simulink model "PE"  (R2024a)
settings: Solver=VariableStepAuto  StartTime=0.0  StopTime=1  RelTol=1e-3
InitFcn:
  | Pe=1/25000
  | w=32.2
  | V=8
  | L=150e-6
  | C=220e-6
  | R=3.2
libraries: spsSeriesRLCBranchLib x5, spsDiodeLib x5, spsMeanLib x2, spsVoltageMeasurementLib x2, spsCurrentMeasurementLib x2, spsIGBTDiodeLib x1, spsACVoltageSourceLib x1, spsDCVoltageSourceLib x1, sps_lib x1
settings Model: Creator=mxf1547  LastModifiedBy=mxf1547

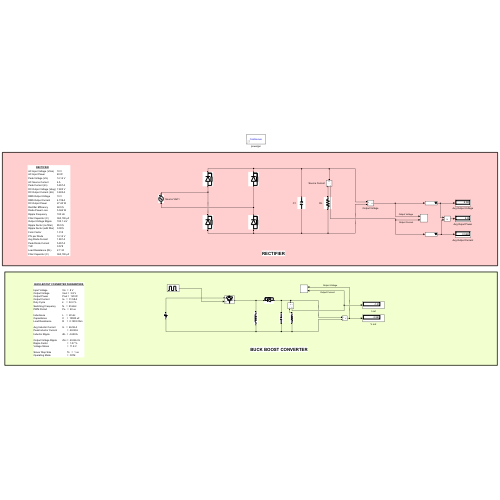
[thumbnail: Simulink's stored preview of the top-level diagram]
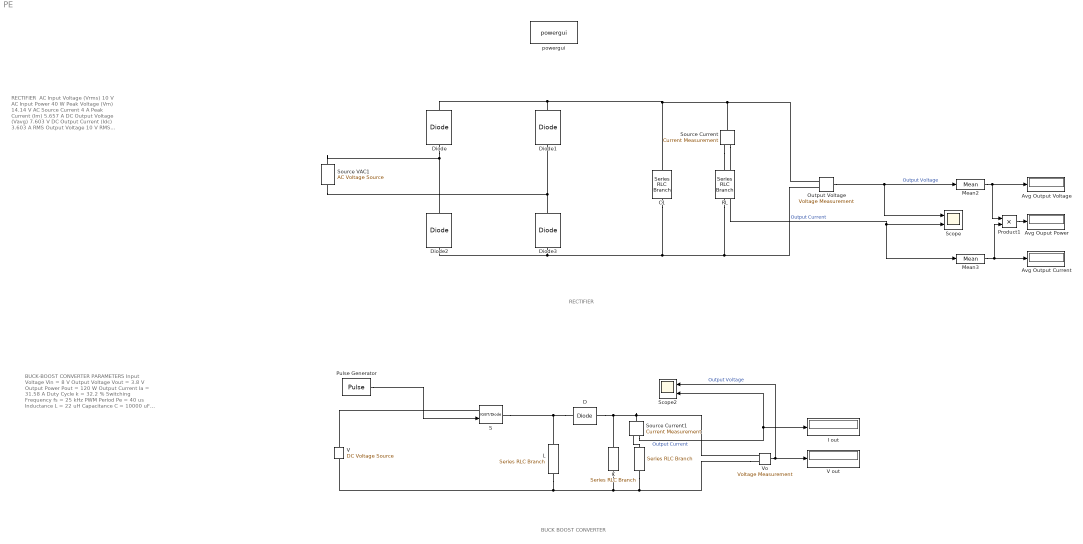
== system PE ==
  note: BUCK-BOOST CONVERTER PARAMETERS
      |
      | Input Voltage Vin = 8 V
      | Output Voltage Vout = 3.8 V
      | Output Power Pout = 120 W
      | Output Current Ia = 31.58 A
      | Duty Cycle k = 32.2 %
      | Switching Frequency fs = 25 kHz
      | PWM Period Pe = 40 us
      |
      | Inductance L = 22 uH
      | Capacitance C = 10000 uF
      | Load Resistance R = 0.1203 Ohm
      |
      | Avg Inductor Current IL = 46.58 A
      | Peak Inductor Current = 48.92 A
      | Inductor Ripple dIL = 4.683 A
      |
      | Output Voltage Ripple dVc = 40.68 mV
      | Ripple Factor = 1.07 %
      | Voltage Stress = 11.8 V
      |
      | Solver Step Size Ts = 1 us
      | Operating Mode = CCM
  note: RECTIFIER
  note: BUCK BOOST CONVERTER
  note: RECTIFIER
      | ​
      |
      | AC Input Voltage (Vrms​)
      | 10 V
      |
      | AC Input Power
      | 40 W
      |
      | Peak Voltage (Vm​)
      | 14.14 V
      |
      | AC Source Current
      | 4 A
      |
      | Peak Current (Im​)
      | 5.657 A
      |
      | DC Output Voltage (Vavg​)
      | 7.603 V
      |
      | DC Output Current (Idc​)
      | 3.603 A
      |
      | RMS Output Voltage
      | 10 V
      |
      | RMS Output Current
      | 4.739 A
      |
      | DC Output Power
      | 27.40 W
      |
      | Rectifier Efficiency
      | 68.5%
      |
      | Diode Power Loss
      | 5.044 W
      |
      | Ripple Frequency
      | 100 Hz
      |
      | Filter Capacitor (C)
      | 360,100 μF
      |
      | Output Voltage Ripple
      | 100.1 mV
      |
      | Ripple Factor (no filter)
      | 85.5%
      |
      | Ripple Factor (with filter)
      | 0.38%
      |
      | Form Factor
      | 1.315
      |
      | PIV per Diode
      | 14.14 V
      |
      | Avg Diode Current
      | 1.801 A
      |
      | Peak Diode Current
      | 5.657 A
      |
      | TUF
      | 0.578
      |
      | Load Resistance (RL​)
      | 2.11 Ω
      |
      | Filter Capacitor (C)
      | 360,100 μF
  " " : spsSeriesRLCBranchLib/Series RLC Branch  LConnTagsString=__new0  RConnTagsString=__new0  BranchType=R  Resistance=R  Inductance=1e-3  SetiL0=off  InitialCurrent=0  Capacitance=1e-6  Setx0=off  InitialVoltage=0  Measurements=None
  Avg Ouput Power : Display
  Avg Output Current : Display
  Avg Output Voltage : Display
  C : spsSeriesRLCBranchLib/Series RLC Branch  LConnTagsString=__new0  RConnTagsString=__new0  BranchType=C  Resistance=1  Inductance=1e-3  SetiL0=off  InitialCurrent=0  Capacitance=C  Setx0=off  InitialVoltage=0  Measurements=None
  C1 : spsSeriesRLCBranchLib/Series RLC Branch  LConnTagsString=__new0  RConnTagsString=__new0  BranchType=C  Resistance=2.11  Inductance=50e-3  SetiL0=off  InitialCurrent=0  Capacitance=360100e-6  Setx0=off  InitialVoltage=0  Measurements=Branch voltage and current
  D : spsDiodeLib/Diode  Ron=0.001  Lon=0  Vf=0.001  IC=0  UseSnubber=off  Rs=500  Cs=250e-9  Measurements=off
  Diode{,1..3} (4 alike) : spsDiodeLib/Diode  Ron=0.001  Lon=0  Vf=0.8  IC=0  UseSnubber=0  Rs=500  Cs=250e-9  Measurements=off
  I out : Display
  L : spsSeriesRLCBranchLib/Series RLC Branch  LConnTagsString=__new0  RConnTagsString=__new0  BranchType=L  Resistance=1  Inductance=L  SetiL0=off  InitialCurrent=0  Capacitance=1e-6  Setx0=off  InitialVoltage=0  Measurements=None
  Mean2 : spsMeanLib/Mean  Freq=50  Vinit=0  Ts=0
  Mean3 : spsMeanLib/Mean  Freq=50  Vinit=0  Ts=0
  Output Voltage : spsVoltageMeasurementLib/Voltage Measurement  PhasorSimulation=off  OutputType=Complex  PSBequivalent=0
  Product1 : Product
  Pulse Generator : DiscretePulseGenerator  PulseType=Time based  Period=Pe  PulseWidth=w
  RL : spsSeriesRLCBranchLib/Series RLC Branch  LConnTagsString=__new0  RConnTagsString=__new0  BranchType=R  Resistance=2.11  Inductance=50e-3  SetiL0=off  InitialCurrent=0  Capacitance=1e-6  Setx0=off  InitialVoltage=0  Measurements=Branch voltage and current
  S : spsIGBTDiodeLib/IGBT//Diode  Ron=1e-3  Rs=1e5  Cs=inf  Measurements=off
  Scope : Scope  NumInputPorts=2
  Scope2 : Scope  NumInputPorts=2
  Source Current : spsCurrentMeasurementLib/Current Measurement  PhasorSimulation=off  OutputType=Complex  PSBequivalent=0
  Source Current1 : spsCurrentMeasurementLib/Current Measurement  PhasorSimulation=off  OutputType=Complex  PSBequivalent=0
  Source VAC1 : spsACVoltageSourceLib/AC Voltage Source  Amplitude=10  Phase=0  Frequency=50  SampleTime=0  Measurements=Voltage  BusType=swing  Pref=10e3  Qref=0  Qmin=-inf  Qmax=+inf
  V : spsDCVoltageSourceLib/DC Voltage Source  Amplitude=V  Measurements=None
  V out : Display
  Vo : spsVoltageMeasurementLib/Voltage Measurement  PhasorSimulation=off  OutputType=Complex  PSBequivalent=0
  powergui : sps_lib/powergui  Priority=1  SimulationMode=Continuous  SampleTime=50e-6  frequency=60  Iterations=50  frequencyindice=0  Pbase=100e6  ErrMax=1e-4  UnitsV=kV  UnitsW=MW  buscounter=0  FunctionMessages=off  echomessages=off  EnableUseOfTLC=off  CurrentSourceSwitches=off  DisableSnubberDevices=off  DisableRonSwitches=off  DisableVfSwitches=off  DisplayEquations=off  AutomaticDiscreteSolvers=off  SolverType=Tustin/Backward Euler (TBE)  Interpol=off  ExternalGateDelay=off  methode=off  Ts=100  x0status=blocks  SPID=on  SwTol=0  HookPort=off  NonlinearTolerance=1e-4  nMaxIteration=100  ContinueOnMaxIteration=off  RestoreLinks=warning  ResistiveCurrentMeasurement=off  Frange=[0:2:500]  Ylog=off  Xlog=on  ShowGrid=off  save=off  variable=ZData  structure=0  ZoomFFT=off  StartTime=0.0  cycles=1  DisplayStyle=1  fundamental=60  FreqAxis=off  MaxFrequency=1000  frequencyindicesteady=1  RmsSteady=1  display=off
  wires:
  Source Current1/1 -> Scope2/2, I out/1  "Output Current"
  Output Voltage/1 -> Mean2/1, Scope/1  "Output Voltage"
  Pulse Generator/1 -> S/1
  Vo/1 -> Scope2/1, V out/1  "Output Voltage"
  Mean3/1 -> Product1/2, Avg Output Current/1
  Product1/1 -> Avg Ouput Power/1
  Mean2/1 -> Avg Output Voltage/1, Product1/1
  Source Current/1 -> Mean3/1, Scope/2  "Output Current"
  connections:
  Diode1/LConn1 -- Source VAC1/LConn1 -- Diode3/RConn1
  Vo/LConn2 -- " "/RConn1 -- C/RConn1 -- L/RConn1 -- V/LConn1
  D/RConn1 -- L/LConn1 -- S/RConn1
  Source Current/LConn1 -- Diode1/RConn1 -- Diode/RConn1 -- C1/LConn1 -- Output Voltage/LConn1
  C/LConn1 -- D/LConn1 -- Vo/LConn1 -- Source Current1/LConn1
  Diode2/LConn1 -- Diode3/LConn1 -- Output Voltage/LConn2 -- RL/RConn1 -- C1/RConn1
  Diode/LConn1 -- Source VAC1/RConn1 -- Diode2/RConn1
  Source Current/RConn1 -- RL/LConn1
  S/LConn1 -- V/RConn1
  Source Current1/RConn1 -- " "/LConn1
